simulink model "GFL_referenceModel"  (R2023b)
settings: Solver=ode23  StartTime=0.0  StopTime=SimulationSetup.Solver.timeSimulationEnd  MaxStep=SimulationSetup.Solver.MaxStep  RelTol=SimulationSetup.Solver.RelTol
undefined symbols (not defined in the file): freq, Ibase, Ki_CC, ki_P, ki_PLL, ki_Q, Kp_CC, kp_P, kp_PLL, kp_Q, Lconv1, Lg, Rconv1, Rg, Sbase, SimulationSetup, Vpeak, wg
libraries: eeStairGenerator x1, spsdq0toabcLib x1
settings Model: Creator=kauchr  LastModifiedBy=kauchr
settings DataIOCC: SaveFinalState=on  SaveOperatingPoint=on  SaveState=on

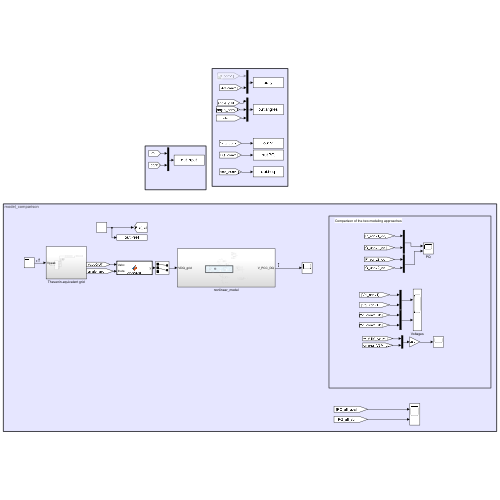
[thumbnail: Simulink's stored preview of the top-level diagram]
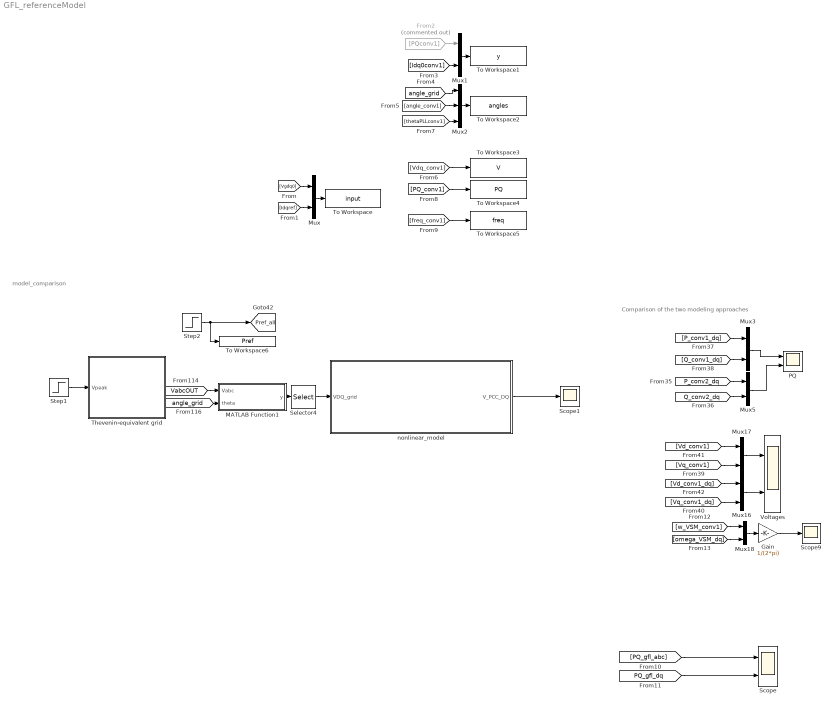
== system GFL_referenceModel ==
  note: model_comparison
  note: Comparison of the two modeling approaches
  From2 : From  Commented=on  GotoTag=PQconv1
  Gain : Gain  Gain=1/(2*pi)
  MATLAB Function1 : MATLAB Function  TreatAsAtomicUnit=on
  Mux{,1,3,5,16..18} (7 alike) : Mux  Inputs=2
  Mux2 : Mux  Inputs=3
  PQ : Scope  NumInputPorts=2
  Scope : Scope  NumInputPorts=2
  Scope1 : Scope
  Scope9 : Scope
  Selector4 : Selector  InputPortWidth=3  IndexOptions=Index vector (dialog)  Indices=[1 2]  OutputSizes=1
  Step1 : Step  Time=SimulationSetup.grid.voltageAmplitudeStep.Time  Before=SimulationSetup.grid.voltageAmplitudeStep.Values(1)  After=SimulationSetup.grid.voltageAmplitudeStep.Values(2)  SampleTime=0
  Step2 : Step  Time=SimulationSetup.converter1.Pref.Time  Before=SimulationSetup.converter1.Pref.Values(1)  After=SimulationSetup.converter1.Pref.Values(2)  SampleTime=0
  Thevenin-equivalent grid : Subsystem
  To Workspace : ToWorkspace  VariableName=input  SaveFormat=Timeseries  SampleTime=-1
  To Workspace1 : ToWorkspace  VariableName=y  SaveFormat=Timeseries  SampleTime=-1
  To Workspace2 : ToWorkspace  VariableName=angles  SaveFormat=Timeseries  SampleTime=-1
  To Workspace3 : ToWorkspace  VariableName=V  SaveFormat=Timeseries  SampleTime=-1
  To Workspace4 : ToWorkspace  VariableName=PQ  SaveFormat=Timeseries  SampleTime=-1
  To Workspace5 : ToWorkspace  VariableName=freq  SaveFormat=Timeseries  SampleTime=-1
  To Workspace6 : ToWorkspace  VariableName=Pref  SaveFormat=Timeseries  SampleTime=-1
  Voltages : Scope  NumInputPorts=2
  nonlinear_model : Subsystem
  tag scope: Pref_all=global
  wires:
  [Vgdq0] -> Mux/1
  [Idqref] -> Mux/2
  Mux/1 -> To Workspace/1
  Mux1/1 -> To Workspace1/1
  From2/1 -> Mux1/1
  [Idq0conv1] -> Mux1/2
  Mux2/1 -> To Workspace2/1
  [angle_grid] -> Mux2/1
  [angle_conv1] -> Mux2/2
  [Vdq_conv1] -> To Workspace3/1
  [thetaPLLconv1] -> Mux2/3
  [PQ_conv1] -> To Workspace4/1
  [freq_conv1] -> To Workspace5/1
  nonlinear_model/1(V_PCC_DQ) -> Scope1/1
  Selector4/1 -> nonlinear_model/1(VDQ_grid)
  [VabcOUT] -> MATLAB Function1/1(Vabc)
  MATLAB Function1/1(y) -> Selector4/1
  [angle_grid] -> MATLAB Function1/2(theta)
  [PQ_gfl_dq] -> Scope/2
  [PQ_gfl_abc] -> Scope/1
  Step2/1 -> To Workspace6/1, [Pref_all]
  [Vq_conv1] -> Mux17/2
  [Vd_conv1_dq] -> Mux16/1
  [Vq_conv1_dq] -> Mux16/2
  [Vd_conv1] -> Mux17/1
  [P_conv1_dq] -> Mux3/1
  [Q_conv1_dq] -> Mux3/2
  Mux5/1 -> PQ/2
  [Q_conv2_dq] -> Mux5/2
  [P_conv2_dq] -> Mux5/1
  Mux3/1 -> PQ/1
  Gain/1 -> Scope9/1
  Mux18/1 -> Gain/1
  [omega_VSM_dq] -> Mux18/2
  [w_VSM_conv1] -> Mux18/1
  Mux17/1 -> Voltages/1
  Mux16/1 -> Voltages/2
  Step1/1 -> Thevenin-equivalent grid/1(Vpeak)

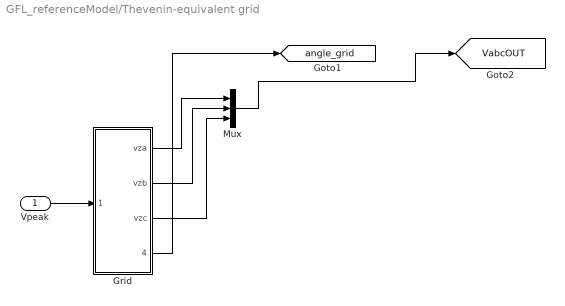
== system GFL_referenceModel/Thevenin-equivalent grid ==
  Vpeak : Inport
  Grid : Subsystem
  Mux : Mux  Inputs=3
  tag scope: VabcOUT=global, angle_grid=global
  wires:
  Grid/4(thetareal) -> [angle_grid]
  Grid/2(vzb) -> Mux/2
  Grid/3(vzc) -> Mux/3
  Mux/1 -> [VabcOUT]
  Grid/1(vza) -> Mux/1
  Vpeak/1 -> Grid/1(Vpeak)

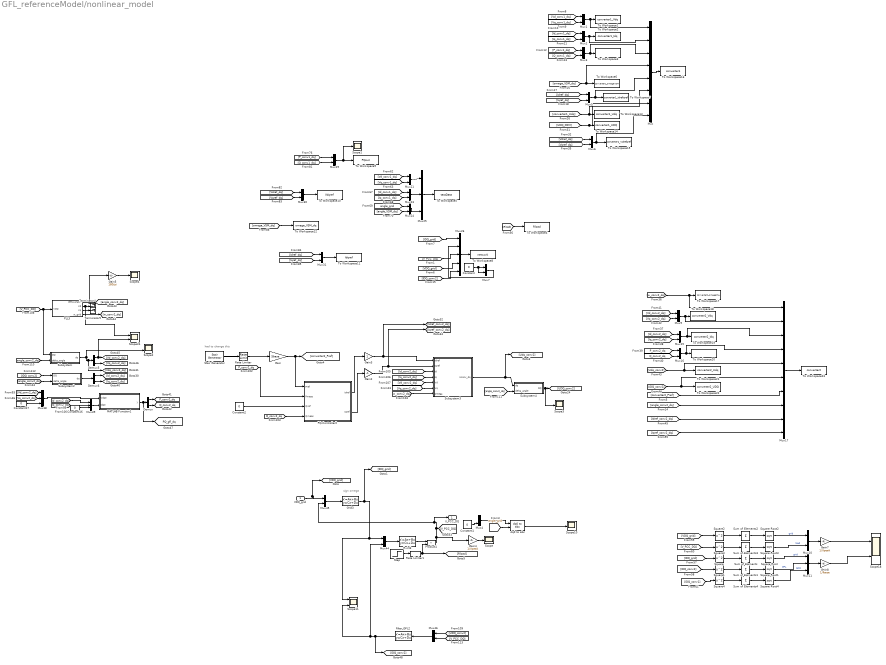
== system GFL_referenceModel/nonlinear_model ==
  note: had to change this
  note: sign omega
  VDQ_grid : Inport
  Constant{,1..2,16..17} (5 alike) : Constant  Value=0
  Demux : Demux  Outputs=2
  Demux5 : Demux  Outputs=2
  Demux6 : Demux  Outputs=2
  Gain : Gain  Gain=Sbase
  Gain2 : Gain  Gain=-1
  Gain3 : Gain
  Gain4 : Gain  Gain=1/Vpeak
  Gain5 : Gain  Gain=180/pi
  Gain7 : Gain  Gain=1/Vpeak
  Gain8 : Gain  Gain=1/Ibase
  Grid3 : StateSpace  A=[-Rg/Lg wg; -wg -Rg/Lg]  B=1/Lg*[eye(2),-eye(2)]  C=eye(2)  D=zeros(2,4)  InitialCondition=0  ContinuousStateAttributes='grid_IDQ'
  MATLAB Function1 : MATLAB Function  TreatAsAtomicUnit=on
  Mux : Mux  Inputs=[2 2 2 1 2 2 2 2]
  Mux{1..3,5..7,9..10,15..16,21,23..24,29..31} (16 alike) : Mux  Inputs=2
  Mux{11,25,38..39} (4 alike) : Mux  Inputs=3
  Mux17 : Mux  Inputs=[1 2 2 2 2 2 1 1 1 1]
  Mux26 : Mux  Inputs=5
  Mux4 : Mux  Inputs=[2 1]
  Mux44 : Mux  Inputs=[2 2]
  Mux45 : Mux  Inputs=[2 2]
  Mux46 : Mux  Inputs=[2 2]
  PLL3 : Subsystem
  PQ-Controller2 : Subsystem
  Product1 : Product
  Rate Limiter : RateLimiter  RisingSlewLimit=100  FallingSlewLimit=-100  SampleTimeMode=inherited
  Rate Limiter1 : RateLimiter  RisingSlewLimit=1000000  FallingSlewLimit=-1000000  SampleTimeMode=inherited
  Rvirt3 : StateSpace  A=[]  B=[]  C=[]  D=[eye(2),eye(2)]  InitialCondition=0  ContinuousStateAttributes='VDQ_PCC'
  Scope{,1,3..4,10} (5 alike) : Scope
  Scope11 : Scope  NumInputPorts=3
  Scope18 : Scope  NumInputPorts=2
  Scope2 : Scope  NumInputPorts=2
  Scope24 : Scope  NumInputPorts=2
  Square{,1..4} (5 alike) : Math  Operator=square
  Square Root{,1..4} (5 alike) : Sqrt
  Stair Generator : eeStairGenerator/Stair Generator  LabelModeActiveChoice=Continuous  TimeInput=SimulationSetup.converter2.Pref.Time  AmplitudeInput=SimulationSetup.converter2.Pref.Values  SampleTime=0  RepeatPattern=off  OutDataTypeStr=double
      settings: LibrarySourceBlock=ee_sl_lib/General Control/Stair Generator
  Step : Step  Time=SimulationSetup.Load.Step.Time  Before=SimulationSetup.Load.Base  After=SimulationSetup.Load.Step.Value  SampleTime=0
  Subsystem : Subsystem
  Subsystem2 : Subsystem
  Subsystem3 : Subsystem
  Subsystem4 : Subsystem
  Sum of Elements{,1..4} (5 alike) : Sum  Inputs=+
  Terminator4 : Terminator
  Terminator5 : Terminator
  To Workspace1 : ToWorkspace  VariableName=converter1_Vdq  SaveFormat=Structure With Time  SampleTime=-1
  To Workspace10 : ToWorkspace  VariableName=Vdqref  SaveFormat=Timeseries  SampleTime=-1
      settings: Save2DSignal=2-D array (concatenate along first dimension)
  To Workspace11 : ToWorkspace  VariableName=Idqref  SaveFormat=Timeseries  SampleTime=-1
      settings: Save2DSignal=2-D array (concatenate along first dimension)
  To Workspace12 : ToWorkspace  VariableName=omega_VSM_dq  SaveFormat=Timeseries  SampleTime=-1
      settings: Save2DSignal=2-D array (concatenate along first dimension)
  To Workspace13 : ToWorkspace  VariableName=converter1_Udq  SaveFormat=Timeseries  SampleTime=-1
      settings: Save2DSignal=2-D array (concatenate along first dimension)
  To Workspace14 : ToWorkspace  VariableName=converter1_UDQ  SaveFormat=Timeseries  SampleTime=-1
      settings: Save2DSignal=2-D array (concatenate along first dimension)
  To Workspace15 : ToWorkspace  VariableName=converter1_Vdrefqref  SaveFormat=Timeseries  SampleTime=-1
      settings: Save2DSignal=2-D array (concatenate along first dimension)
  To Workspace16 : ToWorkspace  VariableName=converter1  SaveFormat=Structure With Time  SampleTime=-1
  To Workspace17 : ToWorkspace  VariableName=converter2_omegaPLL  SaveFormat=Timeseries  SampleTime=-1
      settings: Save2DSignal=2-D array (concatenate along first dimension)
  To Workspace18 : ToWorkspace  VariableName=converter2_Vdq  SaveFormat=Structure With Time  SampleTime=-1
  To Workspace19 : ToWorkspace  VariableName=converter2_Idq  SaveFormat=Structure With Time  SampleTime=-1
  To Workspace2 : ToWorkspace  VariableName=converter1_Idq  SaveFormat=Structure With Time  SampleTime=-1
  To Workspace20 : ToWorkspace  VariableName=converter2_PmeasQmeas  SaveFormat=Structure With Time  SampleTime=-1
  To Workspace21 : ToWorkspace  VariableName=converter2_Udq  SaveFormat=Timeseries  SampleTime=-1
      settings: Save2DSignal=2-D array (concatenate along first dimension)
  To Workspace22 : ToWorkspace  VariableName=converter2_UDQ  SaveFormat=Timeseries  SampleTime=-1
      settings: Save2DSignal=2-D array (concatenate along first dimension)
  To Workspace23 : ToWorkspace  VariableName=converter2  SaveFormat=Structure  SampleTime=-1
      settings: Save2DSignal=2-D array (concatenate along first dimension)
  To Workspace3 : ToWorkspace  VariableName=converter1_PmeasQmeas  SaveFormat=Structure With Time  SampleTime=-1
  To Workspace4 : ToWorkspace  VariableName=Rload  SaveFormat=Timeseries  SampleTime=-1
      settings: Save2DSignal=2-D array (concatenate along first dimension)
  To Workspace5 : ToWorkspace  VariableName=testData  SaveFormat=Structure With Time  SampleTime=-1
  To Workspace6 : ToWorkspace  VariableName=converter1_omegaVSM  SaveFormat=Timeseries  SampleTime=-1
      settings: Save2DSignal=2-D array (concatenate along first dimension)
  To Workspace7 : ToWorkspace  VariableName=converter1_IdrefIqref  SaveFormat=Timeseries  SampleTime=-1
      settings: Save2DSignal=2-D array (concatenate along first dimension)
  To Workspace8 : ToWorkspace  VariableName=network  SaveFormat=Timeseries  SampleTime=-1
      settings: Save2DSignal=2-D array (concatenate along first dimension)
  To Workspace9 : ToWorkspace  VariableName=PQout  SaveFormat=Timeseries  SampleTime=-1
      settings: Save2DSignal=2-D array (concatenate along first dimension)
  dq0 to abc : spsdq0toabcLib/dq0 to abc  Alignment=90 degrees behind phase A axis
  filter_GFL2 : StateSpace  A=[-Rconv1/Lconv1 wg; -wg -Rconv1/Lconv1]  B=1/Lconv1*[eye(2),-eye(2)]  C=eye(2)  D=zeros(2,4)  InitialCondition=0  ContinuousStateAttributes='converter2_IDQ'
  V_PCC_DQ : Outport
  tag scope: PQ_gfl_dq=global, P_conv2_dq=global, Q_conv2_dq=global
  wires:
  Mux24/1 -> Mux25/3
  Mux29/1 -> Scope1/1, To Workspace9/1
  Mux30/1 -> To Workspace10/1
  [Iq_conv1_dq] -> Mux23/2
  [angle_VSM_dq] -> Mux24/2
  Mux31/1 -> To Workspace11/1
  [Q_conv1_dq] -> Mux29/2
  [Vq_conv1_dq] -> Mux21/2
  [Iqref_dq] -> Mux31/2
  [Vdref_dq] -> Mux30/1
  [omega_VSM_dq] -> To Workspace12/1
  Mux23/1 -> Mux25/2
  [angle_grid] -> Mux24/1
  [Id_conv1_dq] -> Mux23/1
  Mux21/1 -> Mux25/1
  [Vd_conv1_dq] -> Mux21/1
  [Idref_dq] -> Mux31/1
  Mux25/1 -> To Workspace5/1
  [Vqref_dq] -> Mux30/2
  [P_conv1_dq] -> Mux29/1
  [Vd_conv2_dq] -> Mux38/1
  Subsystem3/1(Uconv_dq) -> Subsystem4/1(dq), [Udq_conv2]
  MATLAB Function1/1(y) -> [PQ_gfl_dq], Demux/1
  Constant17/1 -> Mux38/3
  Mux38/1 -> MATLAB Function1/1(Vdq0)
  PLL3/2(Vd) -> Scope24/1, Terminator4/1
  Demux6/1 -> [Id_conv2_dq]
  Demux5/2 -> [Vq_conv2_dq]
  [P_conv2_dq] -> PQ-Controller2/2(Pmeas)
  Constant16/1 -> Mux39/3
  Subsystem/1(dq) -> [Vdq_conv2_dq], Demux5/1, Scope2/2
  PLL3/1(delta angle) -> Gain5/1, [angle_conv2_dq]
  [Id_conv2_dq] -> Subsystem3/3(Id)
  [Vq_conv2_dq] -> Mux38/2
  [Id_conv2_dq] -> Mux39/1
  [Iq_conv2_dq] -> Mux39/2
  [V_PCC_DQ] -> Subsystem/1(DQ), PLL3/1(VDQ)
  [Iq_conv2_dq] -> Subsystem3/4(Iq)
  [Q_conv2_dq] -> PQ-Controller2/4(Qmeas)
  PLL3/3(Vq) -> Terminator5/1
  [Vd_conv2_dq] -> Subsystem3/5(Vd)
  [angle_conv2_dq] -> Subsystem/2(delta_angle)
  [Vq_conv2_dq] -> Subsystem3/6(Vq)
  Demux5/1 -> Scope24/2, [Vd_conv2_dq]
  PLL3/4(w_grid) -> [w_conv2_dq]
  Demux6/2 -> [Iq_conv2_dq]
  Mux39/1 -> MATLAB Function1/2(Idq0)
  Mux45/1 -> Grid3/1
  [V_PCC_DQ] -> Mux46/2
  [UDQ_conv2] -> Mux46/1
  Grid3/1 -> [IDQ_grid], Scope11/1, Mux44/1
  Mux46/1 -> filter_GFL2/1
  Mux44/1 -> Rvirt3/1
  [w_conv2_dq] -> Subsystem3/7(omega)
  Mux26/1 -> To Workspace8/1
  [V_PCC_DQ] -> Mux26/3
  [VDQ_grid] -> Mux26/4
  [IDQ_grid] -> Mux26/1
  Mux1/1 -> Mux/1, To Workspace1/1
  [Vq_conv1_dq] -> Mux1/2
  [Vd_conv1_dq] -> Mux1/1
  [Iq_conv1_dq] -> Mux2/2
  [Id_conv1_dq] -> Mux2/1
  Mux3/1 -> Mux/3, To Workspace3/1
  [Q_conv1_dq] -> Mux3/2
  [P_conv1_dq] -> Mux3/1
  [omega_VSM_dq] -> Mux/4, To Workspace6/1
  [Idref_dq] -> Mux5/1
  [Iqref_dq] -> Mux5/2
  Mux5/1 -> Mux/5, To Workspace7/1
  [converter1_Udq] -> Mux/6, To Workspace13/1
  [UDQ_GFM] -> Mux/7, To Workspace14/1
  Mux6/1 -> Mux/8, To Workspace15/1
  [Vqref_dq] -> Mux6/2
  [Vdref_dq] -> Mux6/1
  Mux2/1 -> Mux/2, To Workspace2/1
  Mux/1 -> To Workspace16/1
  [w_conv2_dq] -> Mux17/1, To Workspace17/1
  [Vd_conv2_dq] -> Mux9/1
  Mux9/1 -> Mux17/2, To Workspace18/1
  Mux15/1 -> Mux17/3, To Workspace19/1
  [P_conv2_dq] -> Mux16/1
  [Vq_conv2_dq] -> Mux9/2
  Mux16/1 -> Mux17/4, To Workspace20/1
  [Q_conv2_dq] -> Mux16/2
  [Iq_conv2_dq] -> Mux15/2
  [Id_conv2_dq] -> Mux15/1
  [Udq_conv2] -> Mux17/5, To Workspace21/1
  [UDQ_conv2] -> Mux17/6, To Workspace22/1
  Mux17/1 -> To Workspace23/1
  VDQ_grid/1 -> [VDQ_grid], Mux45/1
  Subsystem2/1(dq) -> Demux6/1
  [angle_conv2_dq] -> Subsystem2/2(delta_angle)
  [IDQ_conv2] -> Subsystem2/1(DQ)
  Subsystem4/1(DQ) -> Scope3/1, [UDQ_conv2]
  [angle_conv2_dq] -> Subsystem4/2(delta_angle)
  Stair Generator/1 -> Rate Limiter/1
  PQ-Controller2/1(Idref) -> Gain3/1
  PQ-Controller2/2(Iqref) -> Gain2/1
  [angle_grid] -> dq0 to abc/2
  Mux4/1 -> dq0 to abc/1
  Constant1/1 -> Mux4/2
  dq0 to abc/1 -> Scope10/1
  Gain3/1 -> [Idref_conv2_dq], Subsystem3/1(Idref)
  Gain2/1 -> Subsystem3/2(Iqref), [Iqref_conv2_dq]
  Gain/1 -> [converter2_Pref], PQ-Controller2/1(Pref)
  Constant2/1 -> PQ-Controller2/3(Qref)
  [converter2_Pref] -> Mux17/7
  Rate Limiter/1 -> Gain/1
  [angle_conv2_dq] -> Mux17/8
  [IDQ_conv2] -> Mux26/5
  filter_GFL2/1 -> Mux44/2, Scope11/3, [IDQ_conv2]
  Constant/1 -> Mux7/2, Mux7/1
  Mux7/1 -> Mux26/2
  [Idref_conv2_dq] -> Mux17/9
  [Iqref_conv2_dq] -> Mux17/10
  Rate Limiter1/1 -> [Rload], Product1/2
  Step/1 -> Rate Limiter1/1
  Rvirt3/1 -> Product1/1
  Product1/1 -> Gain4/1, [V_PCC_DQ], V_PCC_DQ/1, Mux45/2
  [Rload] -> To Workspace4/1
  Gain4/1 -> Scope/1
  Gain5/1 -> Scope4/1
  Square Root4/1 -> Mux11/3  "GFM"
  Square Root3/1 -> Mux10/2  "load"
  Sum of Elements4/1 -> Square Root4/1
  Square4/1 -> Sum of Elements4/1
  [IDQ_conv1] -> Square4/1
  Square/1 -> Sum of Elements/1
  [VDQ_grid] -> Square2/1
  [IDQ_conv2] -> Square1/1
  Mux10/1 -> Gain7/1
  Sum of Elements/1 -> Square Root/1
  Sum of Elements1/1 -> Square Root1/1
  Mux11/1 -> Gain8/1
  Square2/1 -> Sum of Elements2/1
  Square3/1 -> Sum of Elements3/1
  [IDQ_grid] -> Square/1
  Sum of Elements2/1 -> Square Root2/1
  Square1/1 -> Sum of Elements1/1
  [V_PCC_DQ] -> Square3/1
  Sum of Elements3/1 -> Square Root3/1
  Gain8/1 -> Scope18/2
  Square Root2/1 -> Mux10/1  "grid"
  Gain7/1 -> Scope18/1
  Square Root/1 -> Mux11/1  "grid"
  Square Root1/1 -> Mux11/2  "GFL"
  Demux/2 -> [Q_conv2_dq]
  Demux/1 -> [P_conv2_dq]

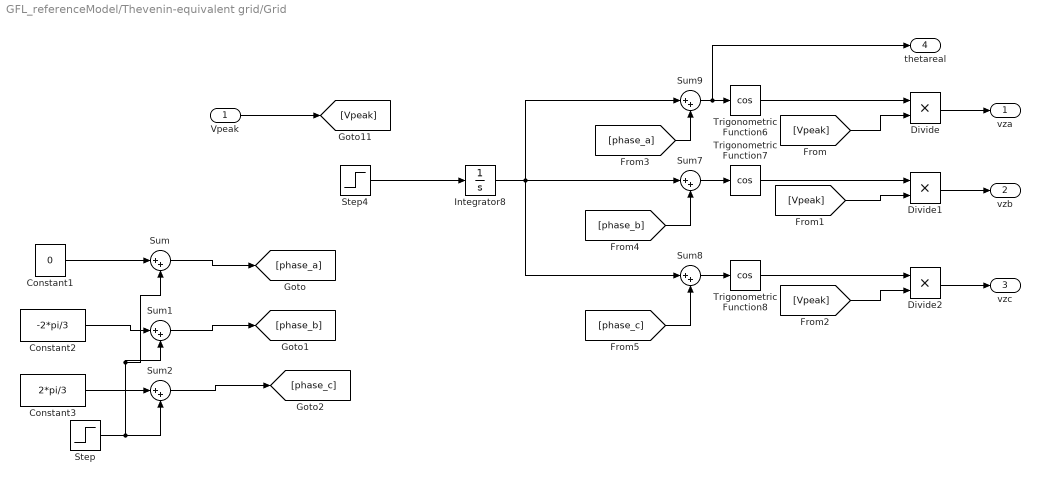
== system GFL_referenceModel/Thevenin-equivalent grid/Grid ==
  Vpeak : Inport
  Constant1 : Constant  Value=0
  Constant2 : Constant  Value=-2*pi/3
  Constant3 : Constant  Value=2*pi/3
  Divide : Product  Inputs=**
  Divide1 : Product  Inputs=**
  Divide2 : Product  Inputs=**
  Integrator8 : Integrator  ContinuousStateAttributes='grid_thetaGRID'
  Step : Step  Time=SimulationSetup.grid.PhaseStep.Time  Before=SimulationSetup.grid.PhaseStep.Values(1)  After=SimulationSetup.grid.PhaseStep.Values(2)  SampleTime=0
  Step4 : Step  Time=SimulationSetup.grid.FrequencyStep.Time  Before=SimulationSetup.grid.FrequencyStep.Values(1)  After=SimulationSetup.grid.FrequencyStep.Values(2)  SampleTime=0
  Sum{,1..2,7..9} (6 alike) : Sum  Inputs=|++
  Trigonometric Function6 : Trigonometry  Operator=cos
  Trigonometric Function7 : Trigonometry  Operator=cos
  Trigonometric Function8 : Trigonometry  Operator=cos
  vza : Outport
  vzb : Outport  Port=2
  vzc : Outport  Port=3
  thetareal : Outport  Port=4
  wires:
  Sum9/1 -> thetareal/1, Trigonometric Function6/1
  [phase_c] -> Sum8/2
  Integrator8/1 -> Sum8/1, Sum9/1, Sum7/1
  [phase_b] -> Sum7/2
  Sum7/1 -> Trigonometric Function7/1
  [phase_a] -> Sum9/2
  Sum8/1 -> Trigonometric Function8/1
  Trigonometric Function6/1 -> Divide/1
  Trigonometric Function7/1 -> Divide1/1
  Trigonometric Function8/1 -> Divide2/1
  Divide/1 -> vza/1
  Divide1/1 -> vzb/1
  Divide2/1 -> vzc/1
  [Vpeak] -> Divide/2
  [Vpeak] -> Divide1/2
  [Vpeak] -> Divide2/2
  Sum1/1 -> [phase_b]
  Sum/1 -> [phase_a]
  Constant1/1 -> Sum/1
  Constant2/1 -> Sum1/1
  Constant3/1 -> Sum2/1
  Sum2/1 -> [phase_c]
  Step/1 -> Sum/2, Sum1/2, Sum2/2
  Step4/1 -> Integrator8/1
  Vpeak/1 -> [Vpeak]

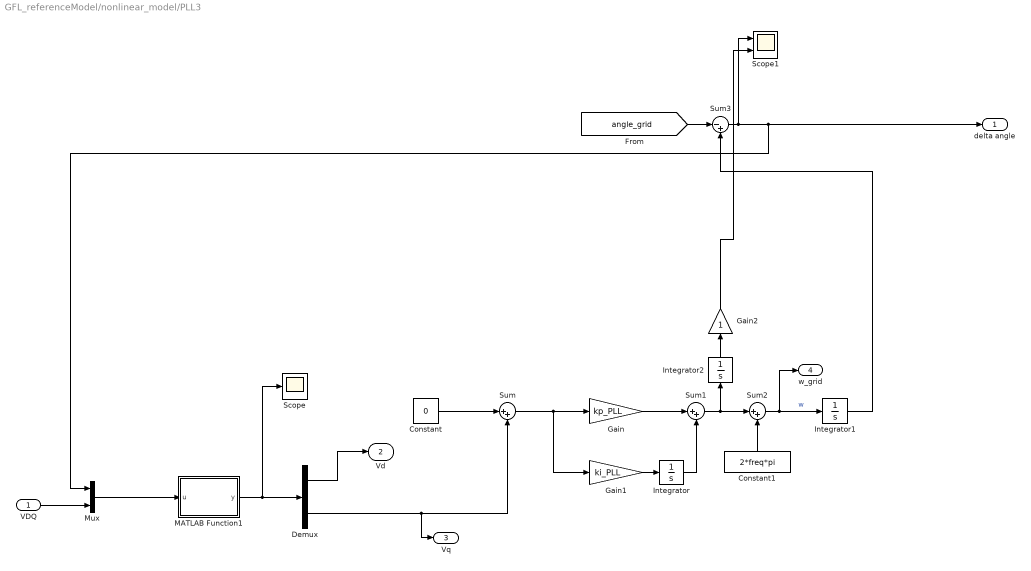
== system GFL_referenceModel/nonlinear_model/PLL3 ==
  VDQ : Inport
  Constant : Constant  Value=0
  Constant1 : Constant  Value=2*freq*pi
  Demux : Demux  Outputs=2
  Gain : Gain  Gain=kp_PLL
  Gain1 : Gain  Gain=ki_PLL
  Gain2 : Gain
  Integrator : Integrator  ContinuousStateAttributes='converter2_xI_PLL'
  Integrator1 : Integrator  ContinuousStateAttributes='converter2_thetaPLL'
  Integrator2 : Integrator  ContinuousStateAttributes='converter2_deltaPLL'
  MATLAB Function1 : MATLAB Function  TreatAsAtomicUnit=on
  Mux : Mux  Inputs=[1 2]
  Scope : Scope
  Scope1 : Scope  NumInputPorts=2
  Sum : Sum  Inputs=|++
  Sum1 : Sum  Inputs=|++
  Sum2 : Sum  Inputs=|++
  Sum3 : Sum  Inputs=|-+
  delta angle : Outport
  Vd : Outport  Port=2
  Vq : Outport  Port=3
  w_grid : Outport  Port=4
  wires:
  Sum1/1 -> Sum2/1, Integrator2/1
  Gain/1 -> Sum1/1
  Integrator/1 -> Sum1/2
  Gain1/1 -> Integrator/1
  Demux/1 -> Vd/1
  Sum2/1 -> w_grid/1, Integrator1/1  "w"
  Constant/1 -> Sum/1
  Constant1/1 -> Sum2/2
  MATLAB Function1/1(y) -> Scope/1, Demux/1
  VDQ/1 -> Mux/2
  Sum/1 -> Gain1/1, Gain/1
  Mux/1 -> MATLAB Function1/1(u)
  Demux/2 -> Vq/1, Sum/2
  [angle_grid] -> Sum3/1
  Integrator1/1 -> Sum3/2
  Integrator2/1 -> Gain2/1
  Sum3/1 -> Scope1/1, Mux/1, delta angle/1
  Gain2/1 -> Scope1/2

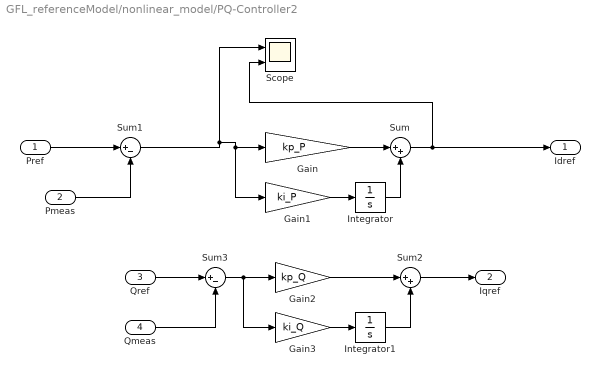
== system GFL_referenceModel/nonlinear_model/PQ-Controller2 ==
  Pref : Inport
  Pmeas : Inport  Port=2
  Qref : Inport  Port=3
  Qmeas : Inport  Port=4
  Gain : Gain  Gain=kp_P
  Gain1 : Gain  Gain=ki_P
  Gain2 : Gain  Gain=kp_Q
  Gain3 : Gain  Gain=ki_Q
  Integrator : Integrator  ContinuousStateAttributes='converter2_xI_Pctrl'
  Integrator1 : Integrator  ContinuousStateAttributes='converter2_xI_Qctrl'
  Scope : Scope  NumInputPorts=2
  Sum : Sum  Inputs=|++
  Sum1 : Sum  Inputs=|+-
  Sum2 : Sum  Inputs=|++
  Sum3 : Sum  Inputs=|+-
  Idref : Outport
  Iqref : Outport  Port=2
  wires:
  Gain1/1 -> Integrator/1
  Integrator/1 -> Sum/2
  Gain/1 -> Sum/1
  Sum/1 -> Idref/1, Scope/2
  Pmeas/1 -> Sum1/2
  Integrator1/1 -> Sum2/2
  Sum2/1 -> Iqref/1
  Sum3/1 -> Gain3/1, Gain2/1
  Gain2/1 -> Sum2/1
  Qmeas/1 -> Sum3/2
  Gain3/1 -> Integrator1/1
  Qref/1 -> Sum3/1
  Sum1/1 -> Scope/1, Gain1/1, Gain/1
  Pref/1 -> Sum1/1

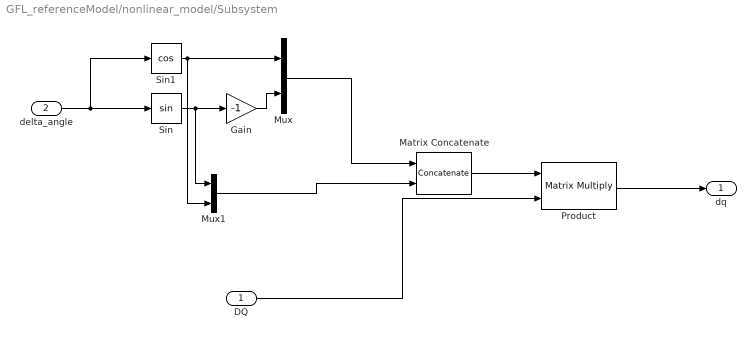
== system GFL_referenceModel/nonlinear_model/Subsystem ==
  DQ : Inport
  delta_angle : Inport  Port=2
  Gain : Gain  Gain=-1
  Matrix Concatenate : Concatenate  Mode=Multidimensional array  ConcatenateDimension=2
  Mux : Mux  Inputs=2
  Mux1 : Mux  Inputs=2
  Product : Product  Multiplication=Matrix(*)
  Sin : Trigonometry
  Sin1 : Trigonometry  Operator=cos
  dq : Outport
  wires:
  Matrix Concatenate/1 -> Product/1
  DQ/1 -> Product/2
  Product/1 -> dq/1
  delta_angle/1 -> Sin1/1, Sin/1
  Sin1/1 -> Mux1/2, Mux/1
  Sin/1 -> Mux1/1, Gain/1
  Gain/1 -> Mux/2
  Mux/1 -> Matrix Concatenate/1
  Mux1/1 -> Matrix Concatenate/2

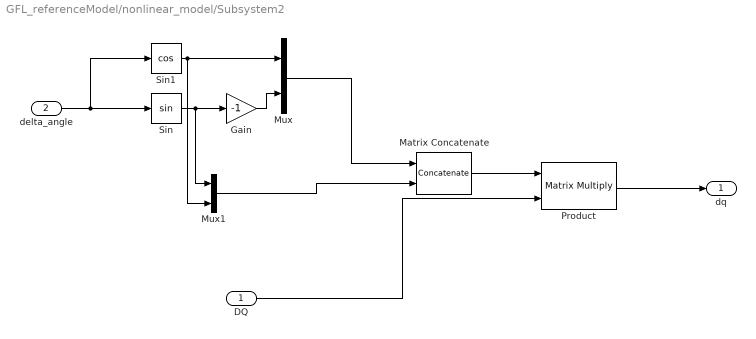
== system GFL_referenceModel/nonlinear_model/Subsystem2 ==
  DQ : Inport
  delta_angle : Inport  Port=2
  Gain : Gain  Gain=-1
  Matrix Concatenate : Concatenate  Mode=Multidimensional array  ConcatenateDimension=2
  Mux : Mux  Inputs=2
  Mux1 : Mux  Inputs=2
  Product : Product  Multiplication=Matrix(*)
  Sin : Trigonometry
  Sin1 : Trigonometry  Operator=cos
  dq : Outport
  wires:
  Matrix Concatenate/1 -> Product/1
  DQ/1 -> Product/2
  Product/1 -> dq/1
  delta_angle/1 -> Sin1/1, Sin/1
  Sin1/1 -> Mux1/2, Mux/1
  Sin/1 -> Mux1/1, Gain/1
  Gain/1 -> Mux/2
  Mux/1 -> Matrix Concatenate/1
  Mux1/1 -> Matrix Concatenate/2

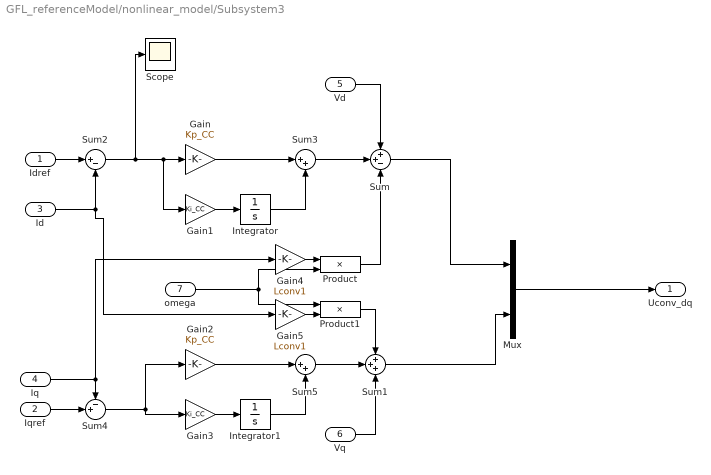
== system GFL_referenceModel/nonlinear_model/Subsystem3 ==
  Idref : Inport
  Iqref : Inport  Port=2
  Id : Inport  Port=3
  Iq : Inport  Port=4
  Vd : Inport  Port=5
  Vq : Inport  Port=6
  omega : Inport  Port=7
  Gain : Gain  Gain=Kp_CC
  Gain1 : Gain  Gain=Ki_CC
  Gain2 : Gain  Gain=Kp_CC
  Gain3 : Gain  Gain=Ki_CC
  Gain4 : Gain  Gain=Lconv1
  Gain5 : Gain  Gain=Lconv1
  Integrator : Integrator  ContinuousStateAttributes='converter2_xId_CC'
  Integrator1 : Integrator  ContinuousStateAttributes='converter2_xIq_CC'
  Mux : Mux  Inputs=2
  Product : Product
  Product1 : Product
  Scope : Scope
  Sum : Sum  Inputs=++-
  Sum1 : Sum  Inputs=+++
  Sum2 : Sum  Inputs=|+-
  Sum3 : Sum  Inputs=|++
  Sum4 : Sum  Inputs=-+|
  Sum5 : Sum  Inputs=|++
  Uconv_dq : Outport
  wires:
  Vd/1 -> Sum/1
  Vq/1 -> Sum1/3
  Sum/1 -> Mux/1
  Sum1/1 -> Mux/2
  Mux/1 -> Uconv_dq/1
  Idref/1 -> Sum2/1
  Id/1 -> Sum2/2, Gain5/1
  Sum2/1 -> Scope/1, Gain1/1, Gain/1
  Gain1/1 -> Integrator/1
  Integrator/1 -> Sum3/2
  Gain/1 -> Sum3/1
  Sum3/1 -> Sum/2
  Iqref/1 -> Sum4/2
  Iq/1 -> Gain4/1, Sum4/1
  Integrator1/1 -> Sum5/2
  Sum5/1 -> Sum1/2
  Gain3/1 -> Integrator1/1
  Gain2/1 -> Sum5/1
  Sum4/1 -> Gain2/1, Gain3/1
  Gain4/1 -> Product/1
  Product/1 -> Sum/3
  omega/1 -> Product/2, Product1/1
  Gain5/1 -> Product1/2
  Product1/1 -> Sum1/1

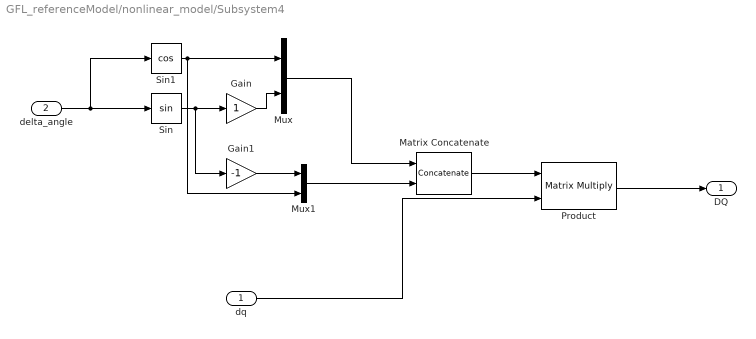
== system GFL_referenceModel/nonlinear_model/Subsystem4 ==
  dq : Inport
  delta_angle : Inport  Port=2
  Gain : Gain
  Gain1 : Gain  Gain=-1
  Matrix Concatenate : Concatenate  Mode=Multidimensional array  ConcatenateDimension=2
  Mux : Mux  Inputs=2
  Mux1 : Mux  Inputs=2
  Product : Product  Multiplication=Matrix(*)
  Sin : Trigonometry
  Sin1 : Trigonometry  Operator=cos
  DQ : Outport
  wires:
  Matrix Concatenate/1 -> Product/1
  dq/1 -> Product/2
  Product/1 -> DQ/1
  delta_angle/1 -> Sin1/1, Sin/1
  Sin1/1 -> Mux1/2, Mux/1
  Sin/1 -> Gain1/1, Gain/1
  Gain/1 -> Mux/2
  Mux/1 -> Matrix Concatenate/1
  Mux1/1 -> Matrix Concatenate/2
  Gain1/1 -> Mux1/1

== matlab function GFL_referenceModel/nonlinear_model/MATLAB Function1 ==
  data: Vdq0 input; y output; Idq0 input
function y = PQcalculation(Vdq0,Idq0)
 % alignment with d-axis
y =3/2*([Vdq0(1)*Idq0(1)+Vdq0(2)*Idq0(2)+2*Vdq0(3)*Idq0(3);Vdq0(2)*Idq0(1)-Vdq0(1)*Idq0(2);]);

== matlab function GFL_referenceModel/nonlinear_model/PLL3/MATLAB Function1 ==
  data: u input; y output
function y = DQ2dq(u)
 
y = inv([cos(u(1)), -sin(u(1)); sin(u(1)), cos(u(1))])*[u(2);u(3)];

== matlab function GFL_referenceModel/MATLAB Function1 ==
  data: Vabc input; y output; theta input
function y = abc2dq0(Vabc,theta)
 % alignment with d-axis
y =2/3*([cos(theta), cos(theta-2*pi/3),cos(theta+2*pi/3); -sin(theta), -sin(theta-2*pi/3), -sin(theta+2*pi/3); sqrt(0.5),sqrt(0.5),sqrt(0.5) ])*[Vabc(1);Vabc(2);Vabc(3)];
